simulink model "Racing_2019"  (R2017a)
settings: Solver=FixedStepDiscrete  StartTime=0.0  StopTime=Inf  FixedStep=1e-3  RelTol=1e-3  EnableMultiTasking=on
PostLoadFcn:
  | , if any(exist('dsrtsu_mdlpostloadfcn', 'file') == [2, 3, 6]), try dsrtsu_mdlpostloadfcn('Execute', bdroot); catch fprintf('Error in PostLoadFcn (dsrtsu_mdlpostloadfcn) for model "%s":\n %s\n', bdroot, lasterr); end, end,
undefined symbols (not defined in the file): Accu_Fans_Enable, Accu_Fans_ON, Accu_Fans_PWM, APPS_Bypass, APPS_Value, AUX_Error_Time, Batt_Temp_High_Threshold, Batt_Temp_Low_Threshold, BMS_Error_Time, BMS_Reset, BMS_Reset_Enable, BMS_Status_Bypass, Brake_Plausibility_Threshold, Brake_Threshold, Brakelight_Test, Braking_Torque, BSPD_State_Bypass, Buzzer, Buzzer_Silent, Buzzer_Test, Calibrate, CAN_Rx_FMEA_Enable, CAN_Status_FMEA_Enable, CAN_Tx_FMEA_Enable, Car_Reset, Car_Reset_Enable, Dash_Fan_PWM, DiscIntNeverNeededParam, DRS_Enable, DRS_PWM_OFF, DRS_PWM_ON, ED_Enable, ED_On, Eject_USB, Enable_Kill, Enable_LED_Test, Fans_Left_Enable, Fans_Left_ON, Fans_Left_PWM, Fans_Right_Enable, Fans_Right_ON, Fans_Right_PWM, I_MAX, IGBT_Temp_High_Threshold, IGBT_Temp_Low_Threshold, Inverter_CAN_Tx_Enable, Inverter_Frequency, KW_Max_Regen_Reset, KW_Max_Reset, LV_DCDC_Temp_High_Threshold, LV_DCDC_Temp_Low_Threshold, magnitude, Plausibility_Bypass, Power_Limiter_Killswitch, Power_Target_kW, Pump_Left_Enable, Pump_Left_ON, Pump_Right_Enable, Pump_Right_ON, Pump_Signal_Left ... (+13)
libraries: rtiusbflightreclib x206, simulink x153, rtican x52, powerlib_meascontrol x47, simulink_extras x17, rti1401lib_adc_type4 x6, rti1401lib_dio_type4 x3, rti1401lib_II_base x1
(part 12 of 23)

== system Racing_2019/Inverter LEFT CAN Rx ==
  note: Error = 1
  Add : Sum
  Air Temp LEFT : Fcn  Expr=0.02*u-216
  Air Temp LEFT Raw : Subsystem  TreatAsAtomicUnit=on
  BTB LEFT Raw : Subsystem  TreatAsAtomicUnit=on
  Commanded Torque LEFT : Subsystem  TreatAsAtomicUnit=on
  Constant : Constant  Value=-32767
  Constant2 : Constant  Value=0
  Data Type Conversion{,4..5,7,9,15..16} (7 alike) : DataTypeConversion  OutDataTypeStr=single
  Data Type Conversion1 : DataTypeConversion  OutDataTypeStr=uint8
  Data Type Conversion{3,6,10,13..14} (5 alike) : DataTypeConversion  OutDataTypeStr=int16
  Data Type Conversion11 : DataTypeConversion  OutDataTypeStr=int8
  Data Type Conversion12 : DataTypeConversion  OutDataTypeStr=int8
  Data Type Conversion2 : DataTypeConversion  OutDataTypeStr=uint8
  Data Type Conversion8 : DataTypeConversion  OutDataTypeStr=uint8
  Edge Detector : powerlib_meascontrol/Logic/Edge Detector  model=Rising  ic=0  Ts=-1
      settings: SourceProductName=Simscape Power Systems  SourceProductBaseCode=PS
  Error LEFT Raw : Subsystem  TreatAsAtomicUnit=on
  Gain : Gain  Gain=0.1
  IGBT Temp LEFT : Fcn  Expr=8.12e-11*u^3-5.61e-6*u^2+0.1361*u-1096
  IGBT Temp LEFT Raw : Subsystem  TreatAsAtomicUnit=on
  IGBT Temp to 10Hz : RateTransition  OutPortSampleTime=1E-1
  "Icont LEFT Raw " : Subsystem  TreatAsAtomicUnit=on
  Inverter_LEFT_CAN_0x181 : Delay  DelayLength=10000  InitialCondition=1  ExternalReset=Level
      settings: InputPortMap=u0,r5
  Inverter_LEFT_CAN_Rx_Counter : Memory  InheritSampleTime=on
  Ipeak LEFT Raw : Subsystem  TreatAsAtomicUnit=on
  Irms LEFT : Gain  Gain=-200/560
  Irms LEFT Raw : Subsystem  TreatAsAtomicUnit=on
  Irms Max LEFT : MinMax  Inputs=2
  LEFT Inverter CAN 0x181 : rtican/RTICAN Receive (RX)   Reserved1=[]  Reserved2=[]  Reserved3=[]  Reserved4=[]  SfcnMessage=[]  Msg_Struct=[]  BoardTypeNo=[]  BoardNo=[]  ChannelNo=[]  Parameters=[]  DialogFcn=[]  UnitName=[]  Revision=[]  UnitValues=[]  DSProperties=struct('RTI',struct('Version',uint32(5),'BlockType',struct('isSLSource',uint8(1),'isSLSink',uint8(1),'isHWSource',uint8(0),'isHWSink',uint8(0),'isSetup',uint8(0),'isInline',uint8(1),'isNonInline',uint8(0),'isInterrupt',uint8(0),'isChannelwise',uint8(0)),'IOBoardType','RTICAN','UnitType','MESSAGE','Identifier','RX','DialogType','MSVC','BlockSet','RTICAN','SlaveProcessor','CAN'))  RTIBlockInterface=struct('OutputPortsWidth',int32([1 1 1]),'OutputPortsActive',[1 1 1],'OutputPortsName',{{'REGID','Value',['RX status']}},'OutputPortsDataType',{{'SS_DOUBLE','SS_DOUBLE','SS_DOUBLE'}},'OutputPortsLabel',{{'REGID','Value',''}},'OutputPortsLabelMode','ON','InputPortsWidth',int32(0),'InputPortsActive',0,'DialogFcn','rtican_message_interface_gui','BlockDisplay',{{'','center'}},'IconTransparency','on','ParameterTunableNames',{{}},'InitLevel',3,'BlockName',struct('Token',{{'CAN_TYPE','_RX_M','_C'}},'BlockParam',{{'BoardTypeNo','BoardNo','ChannelNo'}}),'SampleTime',{{0.001}},'TriggerPort',{{'none'}},'EnablePort',{{'none'}})  RTIBlockParameters=struct('BoardTypeNo',{{1,'OFF',[]}},'BoardNo',{{1,'ON',[1 16]}},'ChannelNo',{{1,'ON',[1 2]}},'Parameters',{{struct('DataFileSupport',struct('DataFileSelectedMaster',0,'DataFileSelectedLocal',0,'DataFileName',['<no datafile support>|'],'DataFileDate','','SelectedFile',['<no file selected>']),'Options',struct('StatusSelected',1,'TimeSelected',0,'DeltaTimeSelected',0,'BytePortSelected',0,'MessageLengthSelected',0,'TriggerPort',struct('Selected',0,'TriggerType',0),'UserCoding',struct('Selected',0,'InterfaceFile','UserDecodingFile','FcnName','UserDecodeFcn','InportSelected',0,'InportWidth',1,'OutportSelected',0,'OutportWidth',1),'EnablePortSelected',0,'SignalOnPortnameSelected',1,'UseRXService',0),'Message',struct('MsgOnBlocknameSelected',0,'MsgName','Inverter_LEFT_Rx','MsgIdFormat',0,'MsgId',385,'MsgLength',4,'NumSignals',2,'SampleTime',0.001,'Signal',struct('SgnName',{'REGID','Value'},'SgnStartBit',{0,8},'SgnLength',{8,16},'SgnType',{0,0},'ModeValue',{-1,-1},'DataType',{0,1},'ByteLayout',{0,0},'Factor',{1,1},'Offset',{0,0},'SgnComment',{{''},{''}},'SgnUnit',{'',''},'Min',{0,0},'Max',{255,255},'SLDataType',{'SS_DOUBLE','SS_DOUBLE'}),'MsgIdNumFormat',1,'MsgComment',{{''}}),'Version',1.2,'general',struct('isFromLib',0)),'OFF',[]}},'GroupId',{{struct('Group',{{'RTICAN'}},'No',1,'Behavior',{{'NAMECHANGE'}},'BlockType',{{'SINK'}},'NameChangeFlag',0),'OFF',[]}},'SFcnRTICANMessage',{{struct('MsgType','RX','SFcnPortType','Scalar','MsgName','Inverter_LEFT_Rx','MsgIdFormat','STD','MsgId',385,'MsgLength',4,'NumSignals',2,'SampleTime',0.001,'Signal',struct('SgnName',{'REGID','Value'},'SgnStartBit',{0,8},'SgnLength',{8,16},'SgnType',{'standard','standard'},'ModeValue',{-1,-1},'DataType',{['unsigned int'],['signed int']},'ByteLayout',{['little endian'],['little endian']},'Factor',{1,1},'Offset',{0,0},'SLDataType',{'SS_DOUBLE','SS_DOUBLE'}),'StatusSelected','yes','TimeSelected','no','DeltaTimeSelected','no','BytePortSelected','no','MessageLengthSelected','no','TriggerPort',struct('Selected','no','TriggerType',0),'UserCoding',struct('Selected','no','InterfaceFile','UserDecodingFile','FcnName','UserDecodeFcn','InportSelected','no','InportWidth',1,'OutportSelected','no','OutportWidth',1),'EnablePortSelected','no','UseRXService','no','BoardType','DS1','BoardNo',1,'ControllerNo',1),'OFF',[]}},'TLCFileName',{{'rtican_rx_message','OFF',[]}})  RTISFcnParameters=struct('SFcnRTICANMessage','struct','TLCFileName','char')  RTIBlockParaDefault=struct('BoardTypeNo',4302,'BoardNo',1,'ChannelNo',1,'Parameters',struct('DataFileSupport',struct('DataFileSelectedMaster',0,'DataFileSelectedLocal',0,'DataFileName','','DataFileDate','','SelectedFile',['<no file selected>']),'Options',struct('StatusSelected',1,'TimeSelected',1,'DeltaTimeSelected',1,'BytePortSelected',0,'MessageLengthSelected',0,'TriggerPort',struct('Selected',0,'TriggerType','rising'),'UserCoding',struct('Selected',0,'InterfaceFile','UserDecodingFile','FcnName','UserDecodeFcn','InportSelected',0,'InportWidth',1,'OutportSelected',0,'OutportWidth',1),'EnablePortSelected',0,'SignalOnPortnameSelected',1,'UseRXService',0),'Message',struct('MsgOnBlocknameSelected',0,'MsgName',['RX Message'],'MsgIdFormat',0,'MsgId',100,'MsgLength',8,'NumSignals',1,'SampleTime',-1,'Signal',struct('SgnName',['RX signal'],'SgnStartBit',0,'SgnLength',8,'SgnType',0,'ModeValue',-1,'DataType',0,'SLDataType','SS_DOUBLE','ByteLayout',0,'Factor',1,'Offset',0,'Min',0,'Max',255,'SgnComment',{{}},'SgnUnit',''),'MsgIdNumFormat',0,'MsgComment',{{''}}),'Version',1.2,'general',struct('isFromLib',1)),'GroupId',struct('Group',{{'RTICAN'}},'No',1,'Behavior',{{'NAMECHANGE'}},'BlockType',{{'SINK'}},'NameChangeFlag',0),'SFcnRTICANMessage',struct('MsgType','RX','MsgName',['RX Message'],'MsgIdFormat','STD','MsgId',100,'MsgLength',8,'NumSignals',1,'SampleTime',-1,'Signal',struct('SgnName',['RX signal'],'SgnStartBit',0,'SgnLength',8,'SgnType','standard','ModeValue',-1,'DataType',['unsigned int'],'ByteLayout',['little endian'],'SLDataType','SS_DOUBLE','Factor',1,'Offset',0),'StatusSelected','yes','TimeSelected','yes','DeltaTimeSelected','yes','BytePortSelected','no','MessageLengthSelected','no','EnablePortSelected','no','UserCoding',struct('Selected','no','InterfaceFile','UserDecodingFile','FcnName','UserDecodeFcn','InportSelected','no','InportWidth',1,'OutportSelected','no','OutportWidth',1),'TriggerPort',struct('Selected','no','TriggerType','rising'),'UseRXService','no','BoardType','DS4302','BoardNo',1,'ControllerNo',1,'SFcnPortType','Scalar'),'TLCFileName','rtican_rx_message')
      settings: AttributesFormatString=Group Id: RTICAN1\n  SourceProductName=dSPACE RTI CAN Blockset
  Motor Power LEFT Raw : Subsystem  TreatAsAtomicUnit=on
  Motor Temp LEFT : Fcn  Expr=0.01746*u-171.5
  Motor Temp LEFT Raw : Subsystem  TreatAsAtomicUnit=on
  Motor Temp to 1Hz : RateTransition  OutPortSampleTime=1
  RPM LEFT : Product  Inputs=**/
  "RPM LEFT Raw " : Subsystem  TreatAsAtomicUnit=on
  RPM Limit LEFT Raw : Subsystem  TreatAsAtomicUnit=on
  Rate Transition : RateTransition  OutPortSampleTime=1e-1
  Rate Transition1 : RateTransition  OutPortSampleTime=1e-1
  Rate Transition2 : RateTransition  OutPortSampleTime=1e-1
  Switch Case : SwitchCase  CaseConditions={32,34,48,73,74,75,77,78,138,143,200,226,246}  ShowDefaultCase=off
  USB_FLIGHT_REC_BL1 : rtiusbflightreclib/USB_FLIGHT_REC_BL1  VarName=Irms_LEFT  DataType=Int16  SampleTime=-1  TLCFileName=rtiusbflightrecwrite  Reserved1=[]  Reserved2=[]  Reserved3=[]  Reserved4=[]  DSProperties=struct('RTI',struct('Version',uint32(3),'BlockType',struct('isSLSource',uint8(0),'isSLSink',uint8(1),'isHWSource',uint8(0),'isHWSink',uint8(0),'isSetup',uint8(0),'isInline',uint8(1),'isNonInline',uint8(0),'isInterrupt',uint8(0),'isChannelwise',uint8(0)),'IOBoardType',{{'DSUSB','FLIGHTREC'}},'UnitType','FLIGHTREC','Identifier','WRITE','DialogType','SL','BlockSet','RTIUSBFLIGHTREC','SlaveProcessor','NONE'))  RTIBlockInterface=struct('InputPortsActive',1,'InputPortsWidth',int32(1),'InputPortsDataType',{{'SS_INT16'}},'BlockDisplay',{{['Write to\nUSB Flight Recorder'],'center'}},'IconTransparency','off','InitLevel',3,'BlockName',struct('Token',{{'USB_FLIGHT_REC_BL1'}}),'MaskDescription',['Write input to the Flight Recorder. Recorded data can be referenced by the specified variable.'],'SampleTime',{{-1}})  RTIBlockParameters=struct('VarName',{{'Irms_LEFT','OFF',[]}},'DataType',{{'Int16','OFF',[]}},'SampleTime',{{-1,'OFF',[]}},'TLCFileName',{{'rtiusbflightrecwrite','OFF',[]}})  RTISFcnParameters=struct('VarName','char','DataType','char','SampleTime','double','TLCFileName','char')  RTIBlockParaDefault=struct('VarName','Var1','DataType','Single','SampleTime',-1,'TLCFileName','rtiusbflightrecwrite')
      settings: SourceProductName=dSPACE RTI USB Flight Rec Blockset
  USB_FLIGHT_REC_BL10 : rtiusbflightreclib/USB_FLIGHT_REC_BL1  VarName=Vout_LEFT  DataType=Single  SampleTime=-1  TLCFileName=rtiusbflightrecwrite  Reserved1=[]  Reserved2=[]  Reserved3=[]  Reserved4=[]  DSProperties=struct('RTI',struct('Version',uint32(3),'BlockType',struct('isSLSource',uint8(0),'isSLSink',uint8(1),'isHWSource',uint8(0),'isHWSink',uint8(0),'isSetup',uint8(0),'isInline',uint8(1),'isNonInline',uint8(0),'isInterrupt',uint8(0),'isChannelwise',uint8(0)),'IOBoardType',{{'DSUSB','FLIGHTREC'}},'UnitType','FLIGHTREC','Identifier','WRITE','DialogType','SL','BlockSet','RTIUSBFLIGHTREC','SlaveProcessor','NONE'))  RTIBlockInterface=struct('InputPortsActive',1,'InputPortsWidth',int32(1),'InputPortsDataType',{{'SS_SINGLE'}},'BlockDisplay',{{['Write to\nUSB Flight Recorder'],'center'}},'IconTransparency','off','InitLevel',3,'BlockName',struct('Token',{{'USB_FLIGHT_REC_BL1'}}),'MaskDescription',['Write input to the Flight Recorder. Recorded data can be referenced by the specified variable.'],'SampleTime',{{-1}})  RTIBlockParameters=struct('VarName',{{'Vout_LEFT','OFF',[]}},'DataType',{{'Single','OFF',[]}},'SampleTime',{{-1,'OFF',[]}},'TLCFileName',{{'rtiusbflightrecwrite','OFF',[]}})  RTISFcnParameters=struct('VarName','char','DataType','char','SampleTime','double','TLCFileName','char')  RTIBlockParaDefault=struct('VarName','Var1','DataType','Single','SampleTime',-1,'TLCFileName','rtiusbflightrecwrite')
      settings: SourceProductName=dSPACE RTI USB Flight Rec Blockset
  USB_FLIGHT_REC_BL2 : rtiusbflightreclib/USB_FLIGHT_REC_BL1  VarName=Motor_Temp_LEFT  DataType=Int16  SampleTime=-1  TLCFileName=rtiusbflightrecwrite  Reserved1=[]  Reserved2=[]  Reserved3=[]  Reserved4=[]  DSProperties=struct('RTI',struct('Version',uint32(3),'BlockType',struct('isSLSource',uint8(0),'isSLSink',uint8(1),'isHWSource',uint8(0),'isHWSink',uint8(0),'isSetup',uint8(0),'isInline',uint8(1),'isNonInline',uint8(0),'isInterrupt',uint8(0),'isChannelwise',uint8(0)),'IOBoardType',{{'DSUSB','FLIGHTREC'}},'UnitType','FLIGHTREC','Identifier','WRITE','DialogType','SL','BlockSet','RTIUSBFLIGHTREC','SlaveProcessor','NONE'))  RTIBlockInterface=struct('InputPortsActive',1,'InputPortsWidth',int32(1),'InputPortsDataType',{{'SS_INT16'}},'BlockDisplay',{{['Write to\nUSB Flight Recorder'],'center'}},'IconTransparency','off','InitLevel',3,'BlockName',struct('Token',{{'USB_FLIGHT_REC_BL1'}}),'MaskDescription',['Write input to the Flight Recorder. Recorded data can be referenced by the specified variable.'],'SampleTime',{{-1}})  RTIBlockParameters=struct('VarName',{{'Motor_Temp_LEFT','OFF',[]}},'DataType',{{'Int16','OFF',[]}},'SampleTime',{{-1,'OFF',[]}},'TLCFileName',{{'rtiusbflightrecwrite','OFF',[]}})  RTISFcnParameters=struct('VarName','char','DataType','char','SampleTime','double','TLCFileName','char')  RTIBlockParaDefault=struct('VarName','Var1','DataType','Single','SampleTime',-1,'TLCFileName','rtiusbflightrecwrite')
      settings: SourceProductName=dSPACE RTI USB Flight Rec Blockset
  USB_FLIGHT_REC_BL3 : rtiusbflightreclib/USB_FLIGHT_REC_BL1  VarName=IGBT_Temp_LEFT  DataType=UInt8  SampleTime=-1  TLCFileName=rtiusbflightrecwrite  Reserved1=[]  Reserved2=[]  Reserved3=[]  Reserved4=[]  DSProperties=struct('RTI',struct('Version',uint32(3),'BlockType',struct('isSLSource',uint8(0),'isSLSink',uint8(1),'isHWSource',uint8(0),'isHWSink',uint8(0),'isSetup',uint8(0),'isInline',uint8(1),'isNonInline',uint8(0),'isInterrupt',uint8(0),'isChannelwise',uint8(0)),'IOBoardType',{{'DSUSB','FLIGHTREC'}},'UnitType','FLIGHTREC','Identifier','WRITE','DialogType','SL','BlockSet','RTIUSBFLIGHTREC','SlaveProcessor','NONE'))  RTIBlockInterface=struct('InputPortsActive',1,'InputPortsWidth',int32(1),'InputPortsDataType',{{'SS_UINT8'}},'BlockDisplay',{{['Write to\nUSB Flight Recorder'],'center'}},'IconTransparency','off','InitLevel',3,'BlockName',struct('Token',{{'USB_FLIGHT_REC_BL1'}}),'MaskDescription',['Write input to the Flight Recorder. Recorded data can be referenced by the specified variable.'],'SampleTime',{{-1}})  RTIBlockParameters=struct('VarName',{{'IGBT_Temp_LEFT','OFF',[]}},'DataType',{{'UInt8','OFF',[]}},'SampleTime',{{-1,'OFF',[]}},'TLCFileName',{{'rtiusbflightrecwrite','OFF',[]}})  RTISFcnParameters=struct('VarName','char','DataType','char','SampleTime','double','TLCFileName','char')  RTIBlockParaDefault=struct('VarName','Var1','DataType','Single','SampleTime',-1,'TLCFileName','rtiusbflightrecwrite')
      settings: SourceProductName=dSPACE RTI USB Flight Rec Blockset
  USB_FLIGHT_REC_BL4 : rtiusbflightreclib/USB_FLIGHT_REC_BL1  VarName=Inverter_Air_Temp_LEFT  DataType=Int16  SampleTime=-1  TLCFileName=rtiusbflightrecwrite  Reserved1=[]  Reserved2=[]  Reserved3=[]  Reserved4=[]  DSProperties=struct('RTI',struct('Version',uint32(3),'BlockType',struct('isSLSource',uint8(0),'isSLSink',uint8(1),'isHWSource',uint8(0),'isHWSink',uint8(0),'isSetup',uint8(0),'isInline',uint8(1),'isNonInline',uint8(0),'isInterrupt',uint8(0),'isChannelwise',uint8(0)),'IOBoardType',{{'DSUSB','FLIGHTREC'}},'UnitType','FLIGHTREC','Identifier','WRITE','DialogType','SL','BlockSet','RTIUSBFLIGHTREC','SlaveProcessor','NONE'))  RTIBlockInterface=struct('InputPortsActive',1,'InputPortsWidth',int32(1),'InputPortsDataType',{{'SS_INT16'}},'BlockDisplay',{{['Write to\nUSB Flight Recorder'],'center'}},'IconTransparency','off','InitLevel',3,'BlockName',struct('Token',{{'USB_FLIGHT_REC_BL1'}}),'MaskDescription',['Write input to the Flight Recorder. Recorded data can be referenced by the specified variable.'],'SampleTime',{{-1}})  RTIBlockParameters=struct('VarName',{{'Inverter_Air_Temp_LEFT','OFF',[]}},'DataType',{{'Int16','OFF',[]}},'SampleTime',{{-1,'OFF',[]}},'TLCFileName',{{'rtiusbflightrecwrite','OFF',[]}})  RTISFcnParameters=struct('VarName','char','DataType','char','SampleTime','double','TLCFileName','char')  RTIBlockParaDefault=struct('VarName','Var1','DataType','Single','SampleTime',-1,'TLCFileName','rtiusbflightrecwrite')
      settings: SourceProductName=dSPACE RTI USB Flight Rec Blockset
  USB_FLIGHT_REC_BL5 : rtiusbflightreclib/USB_FLIGHT_REC_BL1  VarName=Inverter_Error_LEFT  DataType=Int8  SampleTime=-1  TLCFileName=rtiusbflightrecwrite  Reserved1=[]  Reserved2=[]  Reserved3=[]  Reserved4=[]  DSProperties=struct('RTI',struct('Version',uint32(3),'BlockType',struct('isSLSource',uint8(0),'isSLSink',uint8(1),'isHWSource',uint8(0),'isHWSink',uint8(0),'isSetup',uint8(0),'isInline',uint8(1),'isNonInline',uint8(0),'isInterrupt',uint8(0),'isChannelwise',uint8(0)),'IOBoardType',{{'DSUSB','FLIGHTREC'}},'UnitType','FLIGHTREC','Identifier','WRITE','DialogType','SL','BlockSet','RTIUSBFLIGHTREC','SlaveProcessor','NONE'))  RTIBlockInterface=struct('InputPortsActive',1,'InputPortsWidth',int32(1),'InputPortsDataType',{{'SS_INT8'}},'BlockDisplay',{{['Write to\nUSB Flight Recorder'],'center'}},'IconTransparency','off','InitLevel',3,'BlockName',struct('Token',{{'USB_FLIGHT_REC_BL1'}}),'MaskDescription',['Write input to the Flight Recorder. Recorded data can be referenced by the specified variable.'],'SampleTime',{{-1}})  RTIBlockParameters=struct('VarName',{{'Inverter_Error_LEFT','OFF',[]}},'DataType',{{'Int8','OFF',[]}},'SampleTime',{{-1,'OFF',[]}},'TLCFileName',{{'rtiusbflightrecwrite','OFF',[]}})  RTISFcnParameters=struct('VarName','char','DataType','char','SampleTime','double','TLCFileName','char')  RTIBlockParaDefault=struct('VarName','Var1','DataType','Single','SampleTime',-1,'TLCFileName','rtiusbflightrecwrite')
      settings: SourceProductName=dSPACE RTI USB Flight Rec Blockset
  USB_FLIGHT_REC_BL6 : rtiusbflightreclib/USB_FLIGHT_REC_BL1  VarName=Inverter_btb_LEFT  DataType=Int8  SampleTime=-1  TLCFileName=rtiusbflightrecwrite  Reserved1=[]  Reserved2=[]  Reserved3=[]  Reserved4=[]  DSProperties=struct('RTI',struct('Version',uint32(3),'BlockType',struct('isSLSource',uint8(0),'isSLSink',uint8(1),'isHWSource',uint8(0),'isHWSink',uint8(0),'isSetup',uint8(0),'isInline',uint8(1),'isNonInline',uint8(0),'isInterrupt',uint8(0),'isChannelwise',uint8(0)),'IOBoardType',{{'DSUSB','FLIGHTREC'}},'UnitType','FLIGHTREC','Identifier','WRITE','DialogType','SL','BlockSet','RTIUSBFLIGHTREC','SlaveProcessor','NONE'))  RTIBlockInterface=struct('InputPortsActive',1,'InputPortsWidth',int32(1),'InputPortsDataType',{{'SS_INT8'}},'BlockDisplay',{{['Write to\nUSB Flight Recorder'],'center'}},'IconTransparency','off','InitLevel',3,'BlockName',struct('Token',{{'USB_FLIGHT_REC_BL1'}}),'MaskDescription',['Write input to the Flight Recorder. Recorded data can be referenced by the specified variable.'],'SampleTime',{{-1}})  RTIBlockParameters=struct('VarName',{{'Inverter_btb_LEFT','OFF',[]}},'DataType',{{'Int8','OFF',[]}},'SampleTime',{{-1,'OFF',[]}},'TLCFileName',{{'rtiusbflightrecwrite','OFF',[]}})  RTISFcnParameters=struct('VarName','char','DataType','char','SampleTime','double','TLCFileName','char')  RTIBlockParaDefault=struct('VarName','Var1','DataType','Single','SampleTime',-1,'TLCFileName','rtiusbflightrecwrite')
      settings: SourceProductName=dSPACE RTI USB Flight Rec Blockset
  USB_FLIGHT_REC_BL7 : rtiusbflightreclib/USB_FLIGHT_REC_BL1  VarName=Motor_Power_LEFT  DataType=Int16  SampleTime=-1  TLCFileName=rtiusbflightrecwrite  Reserved1=[]  Reserved2=[]  Reserved3=[]  Reserved4=[]  DSProperties=struct('RTI',struct('Version',uint32(3),'BlockType',struct('isSLSource',uint8(0),'isSLSink',uint8(1),'isHWSource',uint8(0),'isHWSink',uint8(0),'isSetup',uint8(0),'isInline',uint8(1),'isNonInline',uint8(0),'isInterrupt',uint8(0),'isChannelwise',uint8(0)),'IOBoardType',{{'DSUSB','FLIGHTREC'}},'UnitType','FLIGHTREC','Identifier','WRITE','DialogType','SL','BlockSet','RTIUSBFLIGHTREC','SlaveProcessor','NONE'))  RTIBlockInterface=struct('InputPortsActive',1,'InputPortsWidth',int32(1),'InputPortsDataType',{{'SS_INT16'}},'BlockDisplay',{{['Write to\nUSB Flight Recorder'],'center'}},'IconTransparency','off','InitLevel',3,'BlockName',struct('Token',{{'USB_FLIGHT_REC_BL1'}}),'MaskDescription',['Write input to the Flight Recorder. Recorded data can be referenced by the specified variable.'],'SampleTime',{{-1}})  RTIBlockParameters=struct('VarName',{{'Motor_Power_LEFT','OFF',[]}},'DataType',{{'Int16','OFF',[]}},'SampleTime',{{-1,'OFF',[]}},'TLCFileName',{{'rtiusbflightrecwrite','OFF',[]}})  RTISFcnParameters=struct('VarName','char','DataType','char','SampleTime','double','TLCFileName','char')  RTIBlockParaDefault=struct('VarName','Var1','DataType','Single','SampleTime',-1,'TLCFileName','rtiusbflightrecwrite')
      settings: SourceProductName=dSPACE RTI USB Flight Rec Blockset
  USB_FLIGHT_REC_BL8 : rtiusbflightreclib/USB_FLIGHT_REC_BL1  VarName=RPM_LEFT  DataType=Int16  SampleTime=-1  TLCFileName=rtiusbflightrecwrite  Reserved1=[]  Reserved2=[]  Reserved3=[]  Reserved4=[]  DSProperties=struct('RTI',struct('Version',uint32(3),'BlockType',struct('isSLSource',uint8(0),'isSLSink',uint8(1),'isHWSource',uint8(0),'isHWSink',uint8(0),'isSetup',uint8(0),'isInline',uint8(1),'isNonInline',uint8(0),'isInterrupt',uint8(0),'isChannelwise',uint8(0)),'IOBoardType',{{'DSUSB','FLIGHTREC'}},'UnitType','FLIGHTREC','Identifier','WRITE','DialogType','SL','BlockSet','RTIUSBFLIGHTREC','SlaveProcessor','NONE'))  RTIBlockInterface=struct('InputPortsActive',1,'InputPortsWidth',int32(1),'InputPortsDataType',{{'SS_INT16'}},'BlockDisplay',{{['Write to\nUSB Flight Recorder'],'center'}},'IconTransparency','off','InitLevel',3,'BlockName',struct('Token',{{'USB_FLIGHT_REC_BL1'}}),'MaskDescription',['Write input to the Flight Recorder. Recorded data can be referenced by the specified variable.'],'SampleTime',{{-1}})  RTIBlockParameters=struct('VarName',{{'RPM_LEFT','OFF',[]}},'DataType',{{'Int16','OFF',[]}},'SampleTime',{{-1,'OFF',[]}},'TLCFileName',{{'rtiusbflightrecwrite','OFF',[]}})  RTISFcnParameters=struct('VarName','char','DataType','char','SampleTime','double','TLCFileName','char')  RTIBlockParaDefault=struct('VarName','Var1','DataType','Single','SampleTime',-1,'TLCFileName','rtiusbflightrecwrite')
      settings: SourceProductName=dSPACE RTI USB Flight Rec Blockset
  USB_FLIGHT_REC_BL9 : rtiusbflightreclib/USB_FLIGHT_REC_BL1  VarName=Commanded_Torque_Left  DataType=Single  SampleTime=-1  TLCFileName=rtiusbflightrecwrite  Reserved1=[]  Reserved2=[]  Reserved3=[]  Reserved4=[]  DSProperties=struct('RTI',struct('Version',uint32(3),'BlockType',struct('isSLSource',uint8(0),'isSLSink',uint8(1),'isHWSource',uint8(0),'isHWSink',uint8(0),'isSetup',uint8(0),'isInline',uint8(1),'isNonInline',uint8(0),'isInterrupt',uint8(0),'isChannelwise',uint8(0)),'IOBoardType',{{'DSUSB','FLIGHTREC'}},'UnitType','FLIGHTREC','Identifier','WRITE','DialogType','SL','BlockSet','RTIUSBFLIGHTREC','SlaveProcessor','NONE'))  RTIBlockInterface=struct('InputPortsActive',1,'InputPortsWidth',int32(1),'InputPortsDataType',{{'SS_SINGLE'}},'BlockDisplay',{{['Write to\nUSB Flight Recorder'],'center'}},'IconTransparency','off','InitLevel',3,'BlockName',struct('Token',{{'USB_FLIGHT_REC_BL1'}}),'MaskDescription',['Write input to the Flight Recorder. Recorded data can be referenced by the specified variable.'],'SampleTime',{{-1}})  RTIBlockParameters=struct('VarName',{{'Commanded_Torque_Left','OFF',[]}},'DataType',{{'Single','OFF',[]}},'SampleTime',{{-1,'OFF',[]}},'TLCFileName',{{'rtiusbflightrecwrite','OFF',[]}})  RTISFcnParameters=struct('VarName','char','DataType','char','SampleTime','double','TLCFileName','char')  RTIBlockParaDefault=struct('VarName','Var1','DataType','Single','SampleTime',-1,'TLCFileName','rtiusbflightrecwrite')
      settings: SourceProductName=dSPACE RTI USB Flight Rec Blockset
  Vout LEFT : Subsystem  TreatAsAtomicUnit=on
  Inverter LEFT CAN Rx Error : Outport
  RPM Left : Outport  Port=2
  IAC Max Left : Outport  Port=3
  IGBT Temp Left : Outport  Port=4
  wires:
  LEFT Inverter CAN 0x181/3 -> Inverter_LEFT_CAN_0x181/2, Edge Detector/1
  Add/1 -> Inverter_LEFT_CAN_Rx_Counter/1
  Data Type Conversion1/1 -> Add/1
  Inverter_LEFT_CAN_Rx_Counter/1 -> Add/2
  Edge Detector/1 -> Data Type Conversion1/1
  Inverter_LEFT_CAN_0x181/1 -> Inverter LEFT CAN Rx Error/1
  Switch Case/1 -> Irms LEFT Raw/Action
  LEFT Inverter CAN 0x181/1 -> Data Type Conversion2/1  "REGID"
  Data Type Conversion2/1 -> Switch Case/1
  Irms LEFT Raw/1(Out1) -> Data Type Conversion/1
  Data Type Conversion/1 -> Irms LEFT/1
  Irms LEFT/1 -> Data Type Conversion3/1
  Data Type Conversion3/1 -> USB_FLIGHT_REC_BL1/1
  "RPM LEFT Raw "/1(Out1) -> Data Type Conversion4/1
  Data Type Conversion4/1 -> RPM LEFT/1
  Constant/1 -> RPM LEFT/3
  Motor Temp LEFT Raw/1(Out1) -> Data Type Conversion5/1
  Data Type Conversion5/1 -> Motor Temp LEFT/1
  Motor Temp LEFT/1 -> Data Type Conversion6/1
  Data Type Conversion6/1 -> Motor Temp to 1Hz/1
  Motor Temp to 1Hz/1 -> USB_FLIGHT_REC_BL2/1
  IGBT Temp LEFT Raw/1(Out1) -> Data Type Conversion7/1
  Data Type Conversion7/1 -> IGBT Temp LEFT/1
  IGBT Temp LEFT/1 -> IGBT Temp to 10Hz/1
  IGBT Temp to 10Hz/1 -> IGBT Temp Left/1, Data Type Conversion8/1
  Data Type Conversion8/1 -> USB_FLIGHT_REC_BL3/1
  Air Temp LEFT Raw/1(Out1) -> Data Type Conversion9/1
  Data Type Conversion9/1 -> Air Temp LEFT/1
  Air Temp LEFT/1 -> Data Type Conversion10/1
  Data Type Conversion10/1 -> USB_FLIGHT_REC_BL4/1
  Ipeak LEFT Raw/1(Out1) -> Irms Max LEFT/1
  "Icont LEFT Raw "/1(Out1) -> Irms Max LEFT/2
  Irms Max LEFT/1 -> Gain/1
  Gain/1 -> IAC Max Left/1
  Error LEFT Raw/1(Out1) -> Data Type Conversion11/1
  Data Type Conversion11/1 -> Rate Transition/1
  Rate Transition/1 -> USB_FLIGHT_REC_BL5/1
  Rate Transition1/1 -> USB_FLIGHT_REC_BL6/1
  Data Type Conversion12/1 -> Rate Transition1/1
  BTB LEFT Raw/1(Out1) -> Data Type Conversion12/1
  Motor Power LEFT Raw/1(Out1) -> Data Type Conversion13/1
  Data Type Conversion13/1 -> Rate Transition2/1
  Rate Transition2/1 -> USB_FLIGHT_REC_BL7/1
  RPM LEFT/1 -> Data Type Conversion14/1
  Data Type Conversion14/1 -> USB_FLIGHT_REC_BL8/1, RPM Left/1
  Constant2/1 -> Inverter_LEFT_CAN_0x181/1
  RPM Limit LEFT Raw/1(Out1) -> RPM LEFT/2
  Switch Case/3 -> "RPM LEFT Raw "/Action
  Switch Case/4 -> Motor Temp LEFT Raw/Action
  Switch Case/5 -> IGBT Temp LEFT Raw/Action
  Switch Case/6 -> Air Temp LEFT Raw/Action
  Switch Case/7 -> Ipeak LEFT Raw/Action
  Switch Case/8 -> "Icont LEFT Raw "/Action
  Commanded Torque LEFT/1(Out1) -> Data Type Conversion15/1
  Data Type Conversion15/1 -> USB_FLIGHT_REC_BL9/1
  Switch Case/2 -> Commanded Torque LEFT/Action
  Vout LEFT/1(Out1) -> Data Type Conversion16/1
  Switch Case/9 -> Vout LEFT/Action
  LEFT Inverter CAN 0x181/2 -> Commanded Torque LEFT/1(In1), Air Temp LEFT Raw/1(In1), Vout LEFT/1(In1), BTB LEFT Raw/1(In1), Motor Power LEFT Raw/1(In1), RPM Limit LEFT Raw/1(In1), Error LEFT Raw/1(In1), "Icont LEFT Raw "/1(In1), Ipeak LEFT Raw/1(In1), IGBT Temp LEFT Raw/1(In1), Motor Temp LEFT Raw/1(In1), "RPM LEFT Raw "/1(In1), Irms LEFT Raw/1(In1)
  Data Type Conversion16/1 -> USB_FLIGHT_REC_BL10/1
  Switch Case/10 -> Error LEFT Raw/Action
  Switch Case/11 -> RPM Limit LEFT Raw/Action
  Switch Case/12 -> BTB LEFT Raw/Action
  Switch Case/13 -> Motor Power LEFT Raw/Action
